simulink model "assignment_2_without_MPPT"  (R2023b)
settings: Solver=VariableStepAuto  StartTime=0.0  StopTime=10  FixedStep=1e-10  MaxStep=1e-4  RelTol=1e-4
values from neighbouring files (symbols this model uses):
  Cdc = 278*10^-3    (= 0.278)    [SOLAR_NEW_MPPT.m]
  fg = 50    [SOLAR_NEW_MPPT.m]
  Ki_cc = Rc/tau_IAC    (= 0.95)    [SOLAR_NEW_MPPT.m]
  Ki_pll = Kp_pll/tau_pll    [SOLAR_NEW_MPPT.m]
  kip = 1/(ki_pq*tau_p)    [SOLAR_NEW_MPPT.m]
  Kiv = w1^2*Cdc    (= 27437.500235)    [SOLAR_NEW_MPPT.m]
  Kp_cc = Lc/tau_IAC    (= 0.03031)    [SOLAR_NEW_MPPT.m]
  Kp_pll = (2*w*e)/Va    [SOLAR_NEW_MPPT.m]
  kpp = tau_IAC/(ki_pq*tau_p)    [SOLAR_NEW_MPPT.m]
  Kpv = 2*e1*w1*Cdc    (= 122.270786078)    [SOLAR_NEW_MPPT.m]
  Lc = 30.31*10^-6    (= 3.031e-05)    [SOLAR_NEW_MPPT.m]
  Rc = 0.95*10^-3    (= 0.00095)    [SOLAR_NEW_MPPT.m]
  Va = sqrt(2)*(Vg/sqrt(3))    [SOLAR_NEW_MPPT.m]
  Vdcn = 1200    [SOLAR_NEW_MPPT.m]
undefined symbols (not defined in the file or in its folder): Io, L, R
libraries: spsControlledVoltageSourceLib x6, slpidlib x6, spsSeriesRLCBranchLib x4, spsControlledCurrentSourceLib x2, spsCurrentMeasurementLib x2, spsGroundLib x1, spsabctodq0Lib x1, spsPower3phInstantaneousLib x1, spsThreePhaseVIMeasurementLib x1, spsVoltageMeasurementLib x1, spspowerguiLib x1
settings Model: Creator=TW  LastModifiedBy=User
settings OptimizationCC: ReuseModelBlockBuffer=off

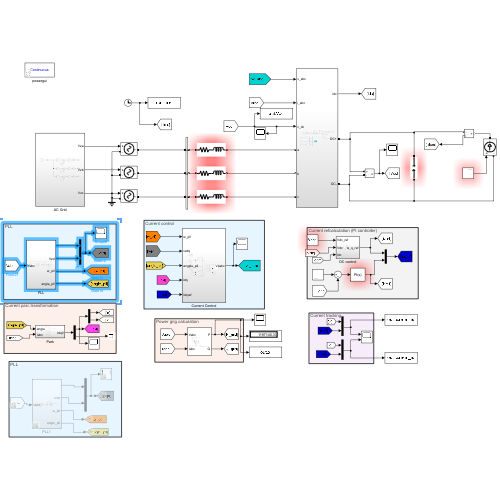
[thumbnail: Simulink's stored preview of the top-level diagram]
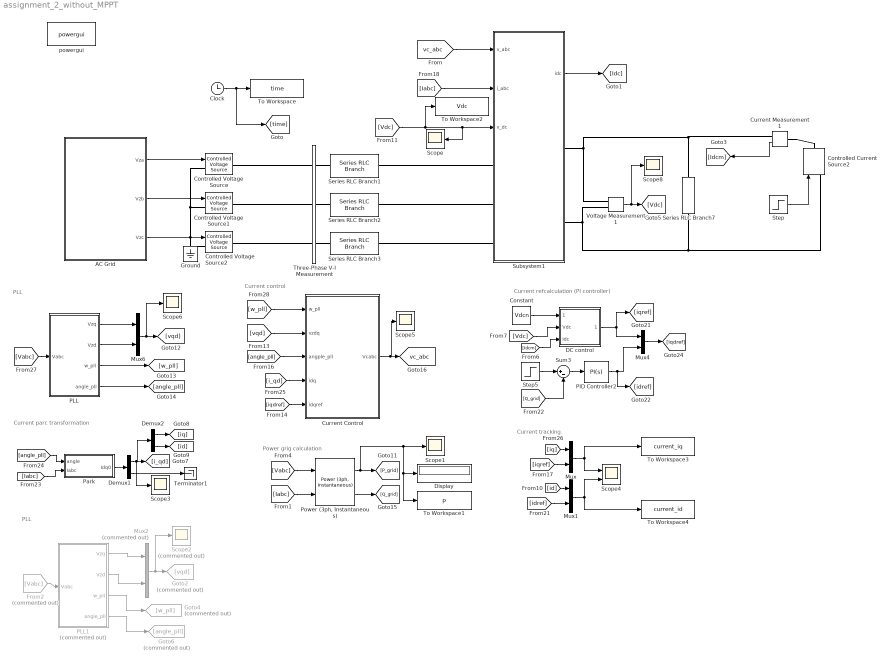
== system assignment_2_without_MPPT ==
  note: Current parc transformation
  note: PLL
  note: Power grig calculation
  note: Current control
  note: Current tracking
  note: Current refcalculation (PI controller)
  note: PLL
  AC Grid : Subsystem
  Clock : Clock
  Constant : Constant  Value=Vdcn
  Controlled Current Source2 : spsControlledCurrentSourceLib/Controlled Current Source  Initialize=on  Source_Type=AC  Amplitude=0  Phase=0  Frequency=0  Measurements=None
  Controlled Voltage Source : spsControlledVoltageSourceLib/Controlled Voltage Source  Initialize=on  Source_Type=AC  Amplitude=0  Phase=0  Frequency=0  Measurements=None
  Controlled Voltage Source1 : spsControlledVoltageSourceLib/Controlled Voltage Source  Initialize=on  Source_Type=AC  Amplitude=0  Phase=0  Frequency=0  Measurements=None
  Controlled Voltage Source2 : spsControlledVoltageSourceLib/Controlled Voltage Source  Initialize=on  Source_Type=AC  Amplitude=0  Phase=0  Frequency=0  Measurements=None
  Current Control : Subsystem
  Current Measurement1 : spsCurrentMeasurementLib/Current Measurement  PhasorSimulation=off  OutputType=Complex  PSBequivalent=0
  DC control : Subsystem
  Demux1 : Demux  Outputs=2
  Demux2 : Demux  Outputs=2
  Display : Display
      settings: Format=bank
  From2 : From  Commented=on  GotoTag=Vabc  TagVisibility=global
  Goto2 : Goto  Commented=on  GotoTag=vqd
  Goto4 : Goto  Commented=on  GotoTag=w_pll
  Goto6 : Goto  Commented=on  GotoTag=angle_pll
  Ground : spsGroundLib/Ground  LConnTagsString=a
  Mux{,1,4,6} (4 alike) : Mux  Inputs=2
  Mux2 : Mux  Commented=on  Inputs=2
  PID Controller2 : slpidlib/PID Controller  Controller=PI  Form=Parallel  TimeDomain=Continuous-time  UseExternalTs=off  SampleTime=-1  IntegratorMethod=Forward Euler  FilterMethod=Forward Euler  ControllerParametersSource=internal  P=kpp  I=kip  UseKiTs=off  D=0  N=100  UseFilter=on  TunerSelectOption=Transfer Function Based (PID Tuner App)  InitialConditionSource=internal  InitialConditionForIntegrator=0  InitialConditionForFilter=0  DifferentiatorICPrevScaledInput=0  ExternalReset=none  TrackingMode=off  Kt=1  LimitOutput=off  SatLimitsSource=internal  UpperSaturationLimit=inf  LowerSaturationLimit=-inf  LinearizeAsGain=on  AntiWindupMode=none  Kb=1  LimitIntegrator=off  UpperIntegratorSaturationLimit=inf  LowerIntegratorSaturationLimit=-inf  POutMin=[]  POutMax=[]  IOutMin=[]  IOutMax=[]  DOutMin=[]  DOutMax=[]  NOutMin=[]  NOutMax=[]  SumOutMin=[]  SumOutMax=[]  SaturationOutMin=[]  SaturationOutMax=[]  PParamMin=[]  PParamMax=[]  IParamMin=[]  IParamMax=[]  DParamMin=[]  DParamMax=[]  NParamMin=[]  NParamMax=[]  KbParamMin=[]  KbParamMax=[]  KtParamMin=[]  KtParamMax=[]  KbOutMin=[]  KbOutMax=[]  KtOutMin=[]  KtOutMax=[]  IntegratorOutMin=[]  IntegratorOutMax=[]  FilterOutMin=[]  FilterOutMax=[]  SumI1OutMin=[]  SumI1OutMax=[]  SumI2OutMin=[]  SumI2OutMax=[]  SumI3OutMin=[]  SumI3OutMax=[]  SumI4OutMin=[]  SumI4OutMax=[]  SumDOutMin=[]  SumDOutMax=[]  DifferentiatorOutMin=[]  DifferentiatorOutMax=[]  FilterDiffOutCoefMin=[]  FilterDiffOutCoefMax=[]  ReciprocalOutMin=[]  ReciprocalOutMax=[]  SumDenOutMin=[]  SumDenOutMax=[]  SumNumOutMin=[]  SumNumOutMax=[]  DivideOutMin=[]  DivideOutMax=[]  UdiffTsProdOutMin=[]  UdiffTsProdOutMax=[]  NTsProdOutMin=[]  NTsProdOutMax=[]  UintegralTsProdOutMin=[]  UintegralTsProdOutMax=[]  UngainTsProdOutMin=[]  UngainTsProdOutMax=[]  ClampingZeroOutDataTypeStr=Inherit: Inherit via back propagation  ClampingZeroOutMin=[]  ClampingZeroOutMax=[]  FilterDenConstantOutDataTypeStr=Inherit: Inherit via back propagation  FilterDenConstantOutMin=[]  FilterDenConstantOutMax=[]  PCopyOutDataTypeStr=Inherit: Inherit via back propagation  PCopyOutMin=[]  PCopyOutMax=[]  NCopyOutDataTypeStr=Inherit: Inherit via back propagation  NCopyOutMin=[]  NCopyOutMax=[]  IntegratorContinuousStateAttributes=''  IntegratorStateMustResolveToSignalObject=off  IntegratorRTWStateStorageClass=Auto  FilterContinuousStateAttributes=''  FilterStateMustResolveToSignalObject=off  FilterRTWStateStorageClass=Auto  ParallelPVariant=InternalParameters  IdealPVariant=Disabled  IVariant=InternalParameters  DVariant=Disabled  IntegratorVariant=Continuous  SatVariant=Disabled  AWVariant=Passthrough  PCopyVariant=Disabled  TRVariant=Disabled  FdbkBlocksVariant=Forward  IdealPFdbkVariant=Disabled  SatFdbkVariant=Disabled  DerivativeFilterVariant=Disabled  NVariant=Disabled  NCopyVariant=Disabled_SignalSpec  FilterICVariant=Disabled  IntegratorICVariant=InternalICs  ExternalResetVariant=Disabled  TRSumVariant=Passthrough  SumFdbkVariant=Disabled  SumVariant=Sum_PI  TsampFilterVariant=InternalTs  TsampNgainVariant=Passthrough  TsampIntegralVariant=Disabled_SignalSpec  ExternalSaturationOutDataTypeStr=Inherit: Same as second input
  PLL : Subsystem
  PLL1 : Subsystem  Commented=on
  Park : Subsystem
  "Power (3ph, Instantaneous)" : spsPower3phInstantaneousLib/Power (3ph, Instantaneous)
  Scope{,1,3,5..6,8} (6 alike) : Scope
  Scope2 : Scope  Commented=on
  Scope4 : Scope  NumInputPorts=2
  Series RLC Branch1 : spsSeriesRLCBranchLib/Series RLC Branch  LConnTagsString=__new0  RConnTagsString=__new0  BranchType=RL  Resistance=Rc  Inductance=Lc  SetiL0=off  InitialCurrent=0  Capacitance=1e-6  Setx0=off  InitialVoltage=0  Measurements=None
  Series RLC Branch2 : spsSeriesRLCBranchLib/Series RLC Branch  LConnTagsString=__new0  RConnTagsString=__new0  BranchType=RL  Resistance=Rc  Inductance=Lc  SetiL0=off  InitialCurrent=0  Capacitance=1e-6  Setx0=off  InitialVoltage=0  Measurements=None
  Series RLC Branch3 : spsSeriesRLCBranchLib/Series RLC Branch  LConnTagsString=__new0  RConnTagsString=__new0  BranchType=RL  Resistance=Rc  Inductance=Lc  SetiL0=off  InitialCurrent=0  Capacitance=1e-6  Setx0=off  InitialVoltage=0  Measurements=None
  Series RLC Branch7 : spsSeriesRLCBranchLib/Series RLC Branch  LConnTagsString=__new0  RConnTagsString=__new0  BranchType=C  Resistance=R  Inductance=L  SetiL0=off  InitialCurrent=0  Capacitance=Cdc  Setx0=on  InitialVoltage=Vdcn  Measurements=None
  Step : Step  After=Io  SampleTime=0
  Step5 : Step  Time=1.5  After=0  SampleTime=0
  Subsystem1 : Subsystem
  Sum3 : Sum  Inputs=|+-
  Terminator1 : Terminator
  Three-Phase V-I Measurement : spsThreePhaseVIMeasurementLib/Three-Phase V-I Measurement  VoltageMeasurement=phase-to-ground  SetLabelV=on  LabelV=Vabc  Vpu=off  VpuLL=off  CurrentMeasurement=yes  SetLabelI=on  LabelI=Iabc  Ipu=off  Pbase=100e6  Vbase=500e3  OutputType=Complex  PhasorSimulation=off  PSBequivalent=0
  To Workspace : ToWorkspace  VariableName=time  SampleTime=-1
  To Workspace1 : ToWorkspace  VariableName=p  SampleTime=-1
  To Workspace2 : ToWorkspace  VariableName=Vdc  SampleTime=-1
  To Workspace3 : ToWorkspace  VariableName=current_iq  SampleTime=-1
  To Workspace4 : ToWorkspace  VariableName=current_id  SampleTime=-1
  Voltage Measurement1 : spsVoltageMeasurementLib/Voltage Measurement  PhasorSimulation=off  OutputType=Complex  PSBequivalent=0
  powergui : spspowerguiLib/powergui  Priority=1  SimulationMode=Continuous  SampleTime=1e-10  frequency=60  Iterations=50  frequencyindice=0  Pbase=100e6  ErrMax=1e-4  UnitsV=kV  UnitsW=MW  buscounter=0  FunctionMessages=off  echomessages=off  EnableUseOfTLC=off  CurrentSourceSwitches=off  DisableSnubberDevices=off  DisableRonSwitches=off  DisableVfSwitches=off  DisplayEquations=off  AutomaticDiscreteSolvers=off  SolverType=Tustin/Backward Euler (TBE)  Interpol=off  ExternalGateDelay=off  methode=off  Ts=100  x0status=blocks  SPID=on  SwTol=0  HookPort=off  NonlinearTolerance=1e-4  nMaxIteration=100  ContinueOnMaxIteration=off  RestoreLinks=warning  ResistiveCurrentMeasurement=off  Frange=[0:2:500]  Ylog=off  Xlog=on  ShowGrid=off  save=off  variable=ZData  structure=0  ZoomFFT=off  StartTime=0.0  cycles=1  DisplayStyle=1  fundamental=60  FreqAxis=off  MaxFrequency=1000  frequencyindicesteady=1  RmsSteady=1  display=off
  tag scope: vc_abc=global
  wires:
  Voltage Measurement1/1 -> Scope8/1, [Vdc]
  Current Measurement1/1 -> [Idcm]
  [Iabc] -> Subsystem1/2(i_abc)
  "Power (3ph, Instantaneous)"/1 -> To Workspace1/1, Display/1, Scope1/1, [P_grid]
  [Vabc] -> "Power (3ph, Instantaneous)"/1
  Demux2/1 -> [iq]
  [angle_pll] -> Current Control/3(angple_pll)
  [i_qd] -> Current Control/4(idq)
  [idref] -> Mux1/2
  [iq] -> Mux/1
  [iqdref] -> Current Control/5(idqref)
  [vqd] -> Current Control/2(vzdq)
  PLL/2(Vzd) -> Mux6/2
  Demux1/1 -> Scope3/1, Demux2/1, [i_qd]
  [iqref] -> Mux/2
  [id] -> Mux1/1
  Demux2/2 -> [id]
  "Power (3ph, Instantaneous)"/2 -> [Q_grid]
  PLL/4(angle_pll) -> [angle_pll]
  [angle_pll] -> Park/1(angle)
  Current Control/1(Vcabc) -> Scope5/1, [vc_abc]
  [w_pll] -> Current Control/1(w_pll)
  Demux1/2 -> Terminator1/1
  [Iabc] -> "Power (3ph, Instantaneous)"/2
  [Iabc] -> Park/2(Iabc)
  Park/1(Idq0) -> Demux1/1
  [Vabc] -> PLL/1(Vabc)
  PLL/1(Vzq) -> Mux6/1
  Mux6/1 -> Scope6/1, [vqd]
  Mux1/1 -> To Workspace4/1, Scope4/2
  PLL/3(w_pll) -> [w_pll]
  Subsystem1/1(idc) -> [Idc]
  [vc_abc] -> Subsystem1/1(v_abc)
  Step/1 -> Controlled Current Source2/1
  [Vdc] -> Subsystem1/3(v_dc), Scope/1, To Workspace2/1
  Clock/1 -> [time], To Workspace/1
  Mux/1 -> To Workspace3/1, Scope4/1
  [Vdc] -> DC control/2(Vdc)
  Sum3/1 -> PID Controller2/1
  Constant/1 -> DC control/1(Vdc_ref)
  [Q_grid] -> Sum3/2
  [Idcm] -> DC control/3(Idc)
  PID Controller2/1 -> [idref], Mux4/2
  Step5/1 -> Sum3/1
  DC control/1(is_q_ref) -> [iqref], Mux4/1
  Mux4/1 -> [iqdref]
  AC Grid/1(Vza) -> Controlled Voltage Source/1
  AC Grid/2(Vzb) -> Controlled Voltage Source1/1
  AC Grid/3(Vzc) -> Controlled Voltage Source2/1
  From2/1 -> PLL1/1(Vabc)
  PLL1/3(w_pll) -> Goto4/1
  PLL1/1(Vzq) -> Mux2/1
  PLL1/2(Vzd) -> Mux2/2
  Mux2/1 -> Scope2/1, Goto2/1
  PLL1/4(angle_pll) -> Goto6/1
  connections:
  Controlled Current Source2/LConn1 -- Subsystem1/RConn2 -- Voltage Measurement1/LConn2 -- Series RLC Branch7/RConn1
  Voltage Measurement1/LConn1 -- Current Measurement1/RConn1 -- Series RLC Branch7/LConn1 -- Subsystem1/RConn1
  Current Measurement1/LConn1 -- Controlled Current Source2/RConn1
  Series RLC Branch1/RConn1 -- Subsystem1/LConn1
  Series RLC Branch3/RConn1 -- Subsystem1/LConn3
  Three-Phase V-I Measurement/LConn3 -- Series RLC Branch3/LConn1
  Series RLC Branch2/RConn1 -- Subsystem1/LConn2
  Three-Phase V-I Measurement/LConn2 -- Series RLC Branch2/LConn1
  Three-Phase V-I Measurement/LConn1 -- Series RLC Branch1/LConn1
  Controlled Voltage Source1/LConn1 -- Controlled Voltage Source/LConn1 -- Controlled Voltage Source2/LConn1 -- Ground/LConn1
  Controlled Voltage Source2/RConn1 -- Three-Phase V-I Measurement/RConn3
  Controlled Voltage Source1/RConn1 -- Three-Phase V-I Measurement/RConn2
  Controlled Voltage Source/RConn1 -- Three-Phase V-I Measurement/RConn1

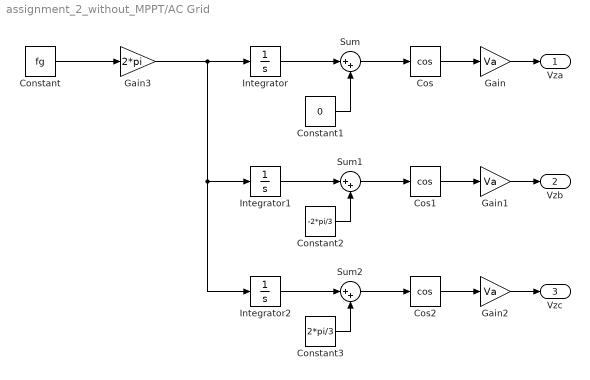
== system assignment_2_without_MPPT/AC Grid ==
  Constant : Constant  Value=fg
  Constant1 : Constant  Value=0
  Constant2 : Constant  Value=-2*pi/3
  Constant3 : Constant  Value=2*pi/3
  Cos : Trigonometry  Operator=cos
  Cos1 : Trigonometry  Operator=cos
  Cos2 : Trigonometry  Operator=cos
  Gain : Gain  Gain=Va
  Gain1 : Gain  Gain=Va
  Gain2 : Gain  Gain=Va
  Gain3 : Gain  Gain=2*pi
  Integrator : Integrator
  Integrator1 : Integrator
  Integrator2 : Integrator
  Sum : Sum  Inputs=|++
  Sum1 : Sum  Inputs=|++
  Sum2 : Sum  Inputs=|++
  Vza : Outport
  Vzb : Outport  Port=2
  Vzc : Outport  Port=3
  wires:
  Integrator2/1 -> Sum2/1
  Cos/1 -> Gain/1
  Gain3/1 -> Integrator1/1, Integrator2/1, Integrator/1
  Integrator1/1 -> Sum1/1
  Cos2/1 -> Gain2/1
  Constant1/1 -> Sum/2
  Gain1/1 -> Vzb/1
  Constant2/1 -> Sum1/2
  Constant3/1 -> Sum2/2
  Gain/1 -> Vza/1
  Sum2/1 -> Cos2/1
  Cos1/1 -> Gain1/1
  Sum/1 -> Cos/1
  Sum1/1 -> Cos1/1
  Gain2/1 -> Vzc/1
  Constant/1 -> Gain3/1
  Integrator/1 -> Sum/1

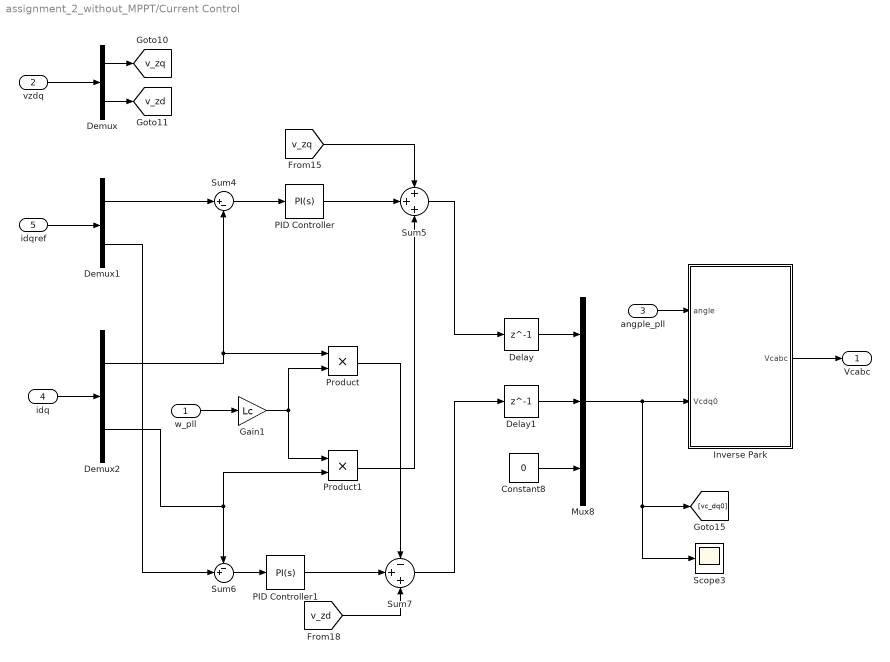
== system assignment_2_without_MPPT/Current Control ==
  w_pll : Inport
  vzdq : Inport  Port=2
  angple_pll : Inport  Port=3
  idq : Inport  Port=4
  idqref : Inport  Port=5
  Constant8 : Constant  Value=0
  Delay : Delay  DelayLength=1
  Delay1 : Delay  DelayLength=1
  Demux : Demux  Outputs=2
  Demux1 : Demux  Outputs=2
  Demux2 : Demux  Outputs=2
  Gain1 : Gain  Gain=Lc
  Inverse Park : Subsystem
  Mux8 : Mux  Inputs=3
  PID Controller : slpidlib/PID Controller  Controller=PI  Form=Parallel  TimeDomain=Continuous-time  UseExternalTs=off  SampleTime=-1  IntegratorMethod=Forward Euler  FilterMethod=Forward Euler  ControllerParametersSource=internal  P=Kp_cc  I=Ki_cc  UseKiTs=off  D=0  N=100  UseFilter=on  TunerSelectOption=Transfer Function Based (PID Tuner App)  InitialConditionSource=internal  InitialConditionForIntegrator=0  InitialConditionForFilter=0  DifferentiatorICPrevScaledInput=0  ExternalReset=none  TrackingMode=off  Kt=1  LimitOutput=off  SatLimitsSource=internal  UpperSaturationLimit=inf  LowerSaturationLimit=-inf  LinearizeAsGain=on  AntiWindupMode=none  Kb=1  LimitIntegrator=off  UpperIntegratorSaturationLimit=inf  LowerIntegratorSaturationLimit=-inf  POutMin=[]  POutMax=[]  IOutMin=[]  IOutMax=[]  DOutMin=[]  DOutMax=[]  NOutMin=[]  NOutMax=[]  SumOutMin=[]  SumOutMax=[]  SaturationOutMin=[]  SaturationOutMax=[]  PParamMin=[]  PParamMax=[]  IParamMin=[]  IParamMax=[]  DParamMin=[]  DParamMax=[]  NParamMin=[]  NParamMax=[]  KbParamMin=[]  KbParamMax=[]  KtParamMin=[]  KtParamMax=[]  KbOutMin=[]  KbOutMax=[]  KtOutMin=[]  KtOutMax=[]  IntegratorOutMin=[]  IntegratorOutMax=[]  FilterOutMin=[]  FilterOutMax=[]  SumI1OutMin=[]  SumI1OutMax=[]  SumI2OutMin=[]  SumI2OutMax=[]  SumI3OutMin=[]  SumI3OutMax=[]  SumI4OutMin=[]  SumI4OutMax=[]  SumDOutMin=[]  SumDOutMax=[]  DifferentiatorOutMin=[]  DifferentiatorOutMax=[]  FilterDiffOutCoefMin=[]  FilterDiffOutCoefMax=[]  ReciprocalOutMin=[]  ReciprocalOutMax=[]  SumDenOutMin=[]  SumDenOutMax=[]  SumNumOutMin=[]  SumNumOutMax=[]  DivideOutMin=[]  DivideOutMax=[]  UdiffTsProdOutMin=[]  UdiffTsProdOutMax=[]  NTsProdOutMin=[]  NTsProdOutMax=[]  UintegralTsProdOutMin=[]  UintegralTsProdOutMax=[]  UngainTsProdOutMin=[]  UngainTsProdOutMax=[]  ClampingZeroOutDataTypeStr=Inherit: Inherit via back propagation  ClampingZeroOutMin=[]  ClampingZeroOutMax=[]  FilterDenConstantOutDataTypeStr=Inherit: Inherit via back propagation  FilterDenConstantOutMin=[]  FilterDenConstantOutMax=[]  PCopyOutDataTypeStr=Inherit: Inherit via back propagation  PCopyOutMin=[]  PCopyOutMax=[]  NCopyOutDataTypeStr=Inherit: Inherit via back propagation  NCopyOutMin=[]  NCopyOutMax=[]  IntegratorContinuousStateAttributes=''  IntegratorStateMustResolveToSignalObject=off  IntegratorRTWStateStorageClass=Auto  FilterContinuousStateAttributes=''  FilterStateMustResolveToSignalObject=off  FilterRTWStateStorageClass=Auto  ParallelPVariant=InternalParameters  IdealPVariant=Disabled  IVariant=InternalParameters  DVariant=Disabled  IntegratorVariant=Continuous  SatVariant=Disabled  AWVariant=Passthrough  PCopyVariant=Disabled  TRVariant=Disabled  FdbkBlocksVariant=Forward  IdealPFdbkVariant=Disabled  SatFdbkVariant=Disabled  DerivativeFilterVariant=Disabled  NVariant=Disabled  NCopyVariant=Disabled_SignalSpec  FilterICVariant=Disabled  IntegratorICVariant=InternalICs  ExternalResetVariant=Disabled  TRSumVariant=Passthrough  SumFdbkVariant=Disabled  SumVariant=Sum_PI  TsampFilterVariant=InternalTs  TsampNgainVariant=Passthrough  TsampIntegralVariant=Disabled_SignalSpec  ExternalSaturationOutDataTypeStr=Inherit: Same as second input
  PID Controller1 : slpidlib/PID Controller  Controller=PI  Form=Parallel  TimeDomain=Continuous-time  UseExternalTs=off  SampleTime=-1  IntegratorMethod=Forward Euler  FilterMethod=Forward Euler  ControllerParametersSource=internal  P=Kp_cc  I=Ki_cc  UseKiTs=off  D=0  N=100  UseFilter=on  TunerSelectOption=Transfer Function Based (PID Tuner App)  InitialConditionSource=internal  InitialConditionForIntegrator=0  InitialConditionForFilter=0  DifferentiatorICPrevScaledInput=0  ExternalReset=none  TrackingMode=off  Kt=1  LimitOutput=off  SatLimitsSource=internal  UpperSaturationLimit=inf  LowerSaturationLimit=-inf  LinearizeAsGain=on  AntiWindupMode=none  Kb=1  LimitIntegrator=off  UpperIntegratorSaturationLimit=inf  LowerIntegratorSaturationLimit=-inf  POutMin=[]  POutMax=[]  IOutMin=[]  IOutMax=[]  DOutMin=[]  DOutMax=[]  NOutMin=[]  NOutMax=[]  SumOutMin=[]  SumOutMax=[]  SaturationOutMin=[]  SaturationOutMax=[]  PParamMin=[]  PParamMax=[]  IParamMin=[]  IParamMax=[]  DParamMin=[]  DParamMax=[]  NParamMin=[]  NParamMax=[]  KbParamMin=[]  KbParamMax=[]  KtParamMin=[]  KtParamMax=[]  KbOutMin=[]  KbOutMax=[]  KtOutMin=[]  KtOutMax=[]  IntegratorOutMin=[]  IntegratorOutMax=[]  FilterOutMin=[]  FilterOutMax=[]  SumI1OutMin=[]  SumI1OutMax=[]  SumI2OutMin=[]  SumI2OutMax=[]  SumI3OutMin=[]  SumI3OutMax=[]  SumI4OutMin=[]  SumI4OutMax=[]  SumDOutMin=[]  SumDOutMax=[]  DifferentiatorOutMin=[]  DifferentiatorOutMax=[]  FilterDiffOutCoefMin=[]  FilterDiffOutCoefMax=[]  ReciprocalOutMin=[]  ReciprocalOutMax=[]  SumDenOutMin=[]  SumDenOutMax=[]  SumNumOutMin=[]  SumNumOutMax=[]  DivideOutMin=[]  DivideOutMax=[]  UdiffTsProdOutMin=[]  UdiffTsProdOutMax=[]  NTsProdOutMin=[]  NTsProdOutMax=[]  UintegralTsProdOutMin=[]  UintegralTsProdOutMax=[]  UngainTsProdOutMin=[]  UngainTsProdOutMax=[]  ClampingZeroOutDataTypeStr=Inherit: Inherit via back propagation  ClampingZeroOutMin=[]  ClampingZeroOutMax=[]  FilterDenConstantOutDataTypeStr=Inherit: Inherit via back propagation  FilterDenConstantOutMin=[]  FilterDenConstantOutMax=[]  PCopyOutDataTypeStr=Inherit: Inherit via back propagation  PCopyOutMin=[]  PCopyOutMax=[]  NCopyOutDataTypeStr=Inherit: Inherit via back propagation  NCopyOutMin=[]  NCopyOutMax=[]  IntegratorContinuousStateAttributes=''  IntegratorStateMustResolveToSignalObject=off  IntegratorRTWStateStorageClass=Auto  FilterContinuousStateAttributes=''  FilterStateMustResolveToSignalObject=off  FilterRTWStateStorageClass=Auto  ParallelPVariant=InternalParameters  IdealPVariant=Disabled  IVariant=InternalParameters  DVariant=Disabled  IntegratorVariant=Continuous  SatVariant=Disabled  AWVariant=Passthrough  PCopyVariant=Disabled  TRVariant=Disabled  FdbkBlocksVariant=Forward  IdealPFdbkVariant=Disabled  SatFdbkVariant=Disabled  DerivativeFilterVariant=Disabled  NVariant=Disabled  NCopyVariant=Disabled_SignalSpec  FilterICVariant=Disabled  IntegratorICVariant=InternalICs  ExternalResetVariant=Disabled  TRSumVariant=Passthrough  SumFdbkVariant=Disabled  SumVariant=Sum_PI  TsampFilterVariant=InternalTs  TsampNgainVariant=Passthrough  TsampIntegralVariant=Disabled_SignalSpec  ExternalSaturationOutDataTypeStr=Inherit: Same as second input
  Product : Product
  Product1 : Product
  Scope3 : Scope
  Sum4 : Sum  Inputs=|+-
  Sum5 : Sum  Inputs=+++
  Sum6 : Sum  Inputs=-+|
  Sum7 : Sum  Inputs=-++
  Vcabc : Outport
  tag scope: v_zd=global, v_zq=global
  wires:
  Demux1/1 -> Sum4/1
  Demux/2 -> [v_zd]
  Sum6/1 -> PID Controller1/1
  PID Controller1/1 -> Sum7/2
  PID Controller/1 -> Sum5/2
  Demux2/1 -> Sum4/2, Product/1
  Mux8/1 -> Scope3/1, [vc_dq0], Inverse Park/2(Vcdq0)
  w_pll/1 -> Gain1/1
  Gain1/1 -> Product1/1, Product/2
  Demux/1 -> [v_zq]
  Demux2/2 -> Sum6/1, Product1/2
  idqref/1 -> Demux1/1
  [v_zd] -> Sum7/3
  Constant8/1 -> Mux8/3
  Demux1/2 -> Sum6/2
  Sum5/1 -> Delay/1
  Delay/1 -> Mux8/1
  [v_zq] -> Sum5/1
  Inverse Park/1(Vcabc) -> Vcabc/1
  Sum4/1 -> PID Controller/1
  Sum7/1 -> Delay1/1
  vzdq/1 -> Demux/1
  Delay1/1 -> Mux8/2
  Product/1 -> Sum7/1
  Product1/1 -> Sum5/3
  angple_pll/1 -> Inverse Park/1(angle)
  idq/1 -> Demux2/1

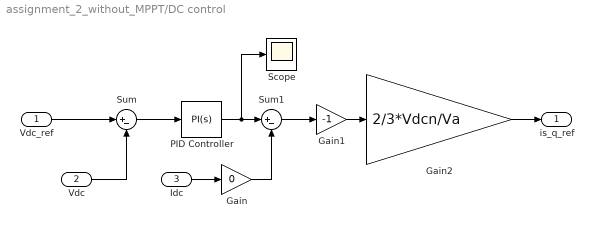
== system assignment_2_without_MPPT/DC control ==
  Vdc_ref : Inport
  Vdc : Inport  Port=2
  Idc : Inport  Port=3
  Gain : Gain  Gain=0
  Gain1 : Gain  Gain=-1
  Gain2 : Gain  Gain=2/3*Vdcn/Va
  PID Controller : slpidlib/PID Controller  Controller=PI  Form=Parallel  TimeDomain=Continuous-time  UseExternalTs=off  SampleTime=-1  IntegratorMethod=Forward Euler  FilterMethod=Forward Euler  ControllerParametersSource=internal  P=Kpv  I=Kiv  UseKiTs=off  D=0  N=100  UseFilter=on  TunerSelectOption=Transfer Function Based (PID Tuner App)  InitialConditionSource=internal  InitialConditionForIntegrator=0  InitialConditionForFilter=0  DifferentiatorICPrevScaledInput=0  ExternalReset=none  TrackingMode=off  Kt=1  LimitOutput=off  SatLimitsSource=internal  UpperSaturationLimit=inf  LowerSaturationLimit=-inf  LinearizeAsGain=on  AntiWindupMode=none  Kb=1  LimitIntegrator=off  UpperIntegratorSaturationLimit=inf  LowerIntegratorSaturationLimit=-inf  POutMin=[]  POutMax=[]  IOutMin=[]  IOutMax=[]  DOutMin=[]  DOutMax=[]  NOutMin=[]  NOutMax=[]  SumOutMin=[]  SumOutMax=[]  SaturationOutMin=[]  SaturationOutMax=[]  PParamMin=[]  PParamMax=[]  IParamMin=[]  IParamMax=[]  DParamMin=[]  DParamMax=[]  NParamMin=[]  NParamMax=[]  KbParamMin=[]  KbParamMax=[]  KtParamMin=[]  KtParamMax=[]  KbOutMin=[]  KbOutMax=[]  KtOutMin=[]  KtOutMax=[]  IntegratorOutMin=[]  IntegratorOutMax=[]  FilterOutMin=[]  FilterOutMax=[]  SumI1OutMin=[]  SumI1OutMax=[]  SumI2OutMin=[]  SumI2OutMax=[]  SumI3OutMin=[]  SumI3OutMax=[]  SumI4OutMin=[]  SumI4OutMax=[]  SumDOutMin=[]  SumDOutMax=[]  DifferentiatorOutMin=[]  DifferentiatorOutMax=[]  FilterDiffOutCoefMin=[]  FilterDiffOutCoefMax=[]  ReciprocalOutMin=[]  ReciprocalOutMax=[]  SumDenOutMin=[]  SumDenOutMax=[]  SumNumOutMin=[]  SumNumOutMax=[]  DivideOutMin=[]  DivideOutMax=[]  UdiffTsProdOutMin=[]  UdiffTsProdOutMax=[]  NTsProdOutMin=[]  NTsProdOutMax=[]  UintegralTsProdOutMin=[]  UintegralTsProdOutMax=[]  UngainTsProdOutMin=[]  UngainTsProdOutMax=[]  ClampingZeroOutDataTypeStr=Inherit: Inherit via back propagation  ClampingZeroOutMin=[]  ClampingZeroOutMax=[]  FilterDenConstantOutDataTypeStr=Inherit: Inherit via back propagation  FilterDenConstantOutMin=[]  FilterDenConstantOutMax=[]  PCopyOutDataTypeStr=Inherit: Inherit via back propagation  PCopyOutMin=[]  PCopyOutMax=[]  NCopyOutDataTypeStr=Inherit: Inherit via back propagation  NCopyOutMin=[]  NCopyOutMax=[]  IntegratorContinuousStateAttributes=''  IntegratorStateMustResolveToSignalObject=off  IntegratorRTWStateStorageClass=Auto  FilterContinuousStateAttributes=''  FilterStateMustResolveToSignalObject=off  FilterRTWStateStorageClass=Auto  ParallelPVariant=InternalParameters  IdealPVariant=Disabled  IVariant=InternalParameters  DVariant=Disabled  IntegratorVariant=Continuous  SatVariant=Disabled  AWVariant=Passthrough  PCopyVariant=Disabled  TRVariant=Disabled  FdbkBlocksVariant=Forward  IdealPFdbkVariant=Disabled  SatFdbkVariant=Disabled  DerivativeFilterVariant=Disabled  NVariant=Disabled  NCopyVariant=Disabled_SignalSpec  FilterICVariant=Disabled  IntegratorICVariant=InternalICs  ExternalResetVariant=Disabled  TRSumVariant=Passthrough  SumFdbkVariant=Disabled  SumVariant=Sum_PI  TsampFilterVariant=InternalTs  TsampNgainVariant=Passthrough  TsampIntegralVariant=Disabled_SignalSpec  ExternalSaturationOutDataTypeStr=Inherit: Same as second input
  Scope : Scope
  Sum : Sum  Inputs=|+-
  Sum1 : Sum  Inputs=|+-
  is_q_ref : Outport
  wires:
  Gain2/1 -> is_q_ref/1
  Sum1/1 -> Gain1/1
  Sum/1 -> PID Controller/1
  Gain1/1 -> Gain2/1
  Gain/1 -> Sum1/2
  Vdc_ref/1 -> Sum/1
  PID Controller/1 -> Sum1/1, Scope/1
  Vdc/1 -> Sum/2
  Idc/1 -> Gain/1

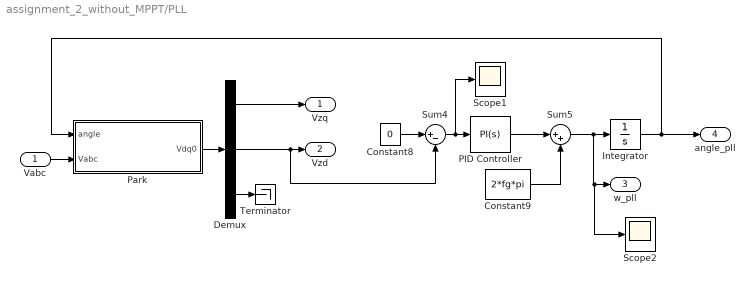
== system assignment_2_without_MPPT/PLL ==
  Vabc : Inport
  Constant8 : Constant  Value=0
  Constant9 : Constant  Value=2*fg*pi
  Demux : Demux  Outputs=3
  Integrator : Integrator
  PID Controller : slpidlib/PID Controller  Controller=PI  Form=Parallel  TimeDomain=Continuous-time  UseExternalTs=off  SampleTime=-1  IntegratorMethod=Forward Euler  FilterMethod=Forward Euler  ControllerParametersSource=internal  P=Kp_pll  I=Ki_pll  UseKiTs=off  D=0  N=100  UseFilter=on  TunerSelectOption=Transfer Function Based (PID Tuner App)  InitialConditionSource=internal  InitialConditionForIntegrator=0  InitialConditionForFilter=0  DifferentiatorICPrevScaledInput=0  ExternalReset=none  TrackingMode=off  Kt=1  LimitOutput=off  SatLimitsSource=internal  UpperSaturationLimit=inf  LowerSaturationLimit=-inf  LinearizeAsGain=on  AntiWindupMode=none  Kb=1  LimitIntegrator=off  UpperIntegratorSaturationLimit=inf  LowerIntegratorSaturationLimit=-inf  POutMin=[]  POutMax=[]  IOutMin=[]  IOutMax=[]  DOutMin=[]  DOutMax=[]  NOutMin=[]  NOutMax=[]  SumOutMin=[]  SumOutMax=[]  SaturationOutMin=[]  SaturationOutMax=[]  PParamMin=[]  PParamMax=[]  IParamMin=[]  IParamMax=[]  DParamMin=[]  DParamMax=[]  NParamMin=[]  NParamMax=[]  KbParamMin=[]  KbParamMax=[]  KtParamMin=[]  KtParamMax=[]  KbOutMin=[]  KbOutMax=[]  KtOutMin=[]  KtOutMax=[]  IntegratorOutMin=[]  IntegratorOutMax=[]  FilterOutMin=[]  FilterOutMax=[]  SumI1OutMin=[]  SumI1OutMax=[]  SumI2OutMin=[]  SumI2OutMax=[]  SumI3OutMin=[]  SumI3OutMax=[]  SumI4OutMin=[]  SumI4OutMax=[]  SumDOutMin=[]  SumDOutMax=[]  DifferentiatorOutMin=[]  DifferentiatorOutMax=[]  FilterDiffOutCoefMin=[]  FilterDiffOutCoefMax=[]  ReciprocalOutMin=[]  ReciprocalOutMax=[]  SumDenOutMin=[]  SumDenOutMax=[]  SumNumOutMin=[]  SumNumOutMax=[]  DivideOutMin=[]  DivideOutMax=[]  UdiffTsProdOutMin=[]  UdiffTsProdOutMax=[]  NTsProdOutMin=[]  NTsProdOutMax=[]  UintegralTsProdOutMin=[]  UintegralTsProdOutMax=[]  UngainTsProdOutMin=[]  UngainTsProdOutMax=[]  ClampingZeroOutDataTypeStr=Inherit: Inherit via back propagation  ClampingZeroOutMin=[]  ClampingZeroOutMax=[]  FilterDenConstantOutDataTypeStr=Inherit: Inherit via back propagation  FilterDenConstantOutMin=[]  FilterDenConstantOutMax=[]  PCopyOutDataTypeStr=Inherit: Inherit via back propagation  PCopyOutMin=[]  PCopyOutMax=[]  NCopyOutDataTypeStr=Inherit: Inherit via back propagation  NCopyOutMin=[]  NCopyOutMax=[]  IntegratorContinuousStateAttributes=''  IntegratorStateMustResolveToSignalObject=off  IntegratorRTWStateStorageClass=Auto  FilterContinuousStateAttributes=''  FilterStateMustResolveToSignalObject=off  FilterRTWStateStorageClass=Auto  ParallelPVariant=InternalParameters  IdealPVariant=Disabled  IVariant=InternalParameters  DVariant=Disabled  IntegratorVariant=Continuous  SatVariant=Disabled  AWVariant=Passthrough  PCopyVariant=Disabled  TRVariant=Disabled  FdbkBlocksVariant=Forward  IdealPFdbkVariant=Disabled  SatFdbkVariant=Disabled  DerivativeFilterVariant=Disabled  NVariant=Disabled  NCopyVariant=Disabled_SignalSpec  FilterICVariant=Disabled  IntegratorICVariant=InternalICs  ExternalResetVariant=Disabled  TRSumVariant=Passthrough  SumFdbkVariant=Disabled  SumVariant=Sum_PI  TsampFilterVariant=InternalTs  TsampNgainVariant=Passthrough  TsampIntegralVariant=Disabled_SignalSpec  ExternalSaturationOutDataTypeStr=Inherit: Same as second input
  Park : Subsystem
  Scope1 : Scope
  Scope2 : Scope
  Sum4 : Sum  Inputs=|+-
  Sum5 : Sum  Inputs=|++
  Terminator : Terminator
  Vzq : Outport
  Vzd : Outport  Port=2
  w_pll : Outport  Port=3
  angle_pll : Outport  Port=4
  wires:
  Vabc/1 -> Park/2(Vabc)
  Constant8/1 -> Sum4/1
  Demux/2 -> Sum4/2, Vzd/1
  PID Controller/1 -> Sum5/1
  Demux/1 -> Vzq/1
  Park/1(Vdq0) -> Demux/1
  Constant9/1 -> Sum5/2
  Integrator/1 -> angle_pll/1, Park/1(angle)
  Demux/3 -> Terminator/1
  Sum5/1 -> Scope2/1, w_pll/1, Integrator/1
  Sum4/1 -> Scope1/1, PID Controller/1

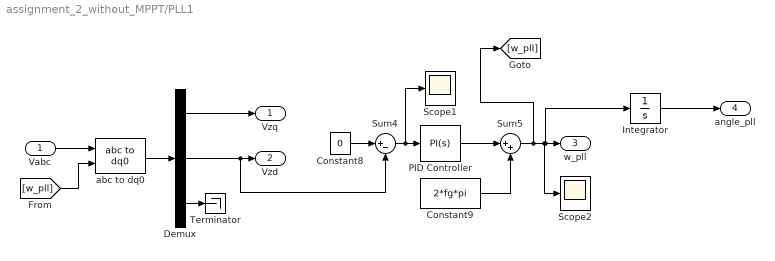
== system assignment_2_without_MPPT/PLL1 ==
  Vabc : Inport
  Constant8 : Constant  Value=0
  Constant9 : Constant  Value=2*fg*pi
  Demux : Demux  Outputs=3
  Integrator : Integrator
  PID Controller : slpidlib/PID Controller  Controller=PI  Form=Parallel  TimeDomain=Continuous-time  UseExternalTs=off  SampleTime=-1  IntegratorMethod=Forward Euler  FilterMethod=Forward Euler  ControllerParametersSource=internal  P=Kp_pll  I=Ki_pll  UseKiTs=off  D=0  N=100  UseFilter=on  TunerSelectOption=Transfer Function Based (PID Tuner App)  InitialConditionSource=internal  InitialConditionForIntegrator=0  InitialConditionForFilter=0  DifferentiatorICPrevScaledInput=0  ExternalReset=none  TrackingMode=off  Kt=1  LimitOutput=off  SatLimitsSource=internal  UpperSaturationLimit=inf  LowerSaturationLimit=-inf  LinearizeAsGain=on  AntiWindupMode=none  Kb=1  LimitIntegrator=off  UpperIntegratorSaturationLimit=inf  LowerIntegratorSaturationLimit=-inf  POutMin=[]  POutMax=[]  IOutMin=[]  IOutMax=[]  DOutMin=[]  DOutMax=[]  NOutMin=[]  NOutMax=[]  SumOutMin=[]  SumOutMax=[]  SaturationOutMin=[]  SaturationOutMax=[]  PParamMin=[]  PParamMax=[]  IParamMin=[]  IParamMax=[]  DParamMin=[]  DParamMax=[]  NParamMin=[]  NParamMax=[]  KbParamMin=[]  KbParamMax=[]  KtParamMin=[]  KtParamMax=[]  KbOutMin=[]  KbOutMax=[]  KtOutMin=[]  KtOutMax=[]  IntegratorOutMin=[]  IntegratorOutMax=[]  FilterOutMin=[]  FilterOutMax=[]  SumI1OutMin=[]  SumI1OutMax=[]  SumI2OutMin=[]  SumI2OutMax=[]  SumI3OutMin=[]  SumI3OutMax=[]  SumI4OutMin=[]  SumI4OutMax=[]  SumDOutMin=[]  SumDOutMax=[]  DifferentiatorOutMin=[]  DifferentiatorOutMax=[]  FilterDiffOutCoefMin=[]  FilterDiffOutCoefMax=[]  ReciprocalOutMin=[]  ReciprocalOutMax=[]  SumDenOutMin=[]  SumDenOutMax=[]  SumNumOutMin=[]  SumNumOutMax=[]  DivideOutMin=[]  DivideOutMax=[]  UdiffTsProdOutMin=[]  UdiffTsProdOutMax=[]  NTsProdOutMin=[]  NTsProdOutMax=[]  UintegralTsProdOutMin=[]  UintegralTsProdOutMax=[]  UngainTsProdOutMin=[]  UngainTsProdOutMax=[]  ClampingZeroOutDataTypeStr=Inherit: Inherit via back propagation  ClampingZeroOutMin=[]  ClampingZeroOutMax=[]  FilterDenConstantOutDataTypeStr=Inherit: Inherit via back propagation  FilterDenConstantOutMin=[]  FilterDenConstantOutMax=[]  PCopyOutDataTypeStr=Inherit: Inherit via back propagation  PCopyOutMin=[]  PCopyOutMax=[]  NCopyOutDataTypeStr=Inherit: Inherit via back propagation  NCopyOutMin=[]  NCopyOutMax=[]  IntegratorContinuousStateAttributes=''  IntegratorStateMustResolveToSignalObject=off  IntegratorRTWStateStorageClass=Auto  FilterContinuousStateAttributes=''  FilterStateMustResolveToSignalObject=off  FilterRTWStateStorageClass=Auto  ParallelPVariant=InternalParameters  IdealPVariant=Disabled  IVariant=InternalParameters  DVariant=Disabled  IntegratorVariant=Continuous  SatVariant=Disabled  AWVariant=Passthrough  PCopyVariant=Disabled  TRVariant=Disabled  FdbkBlocksVariant=Forward  IdealPFdbkVariant=Disabled  SatFdbkVariant=Disabled  DerivativeFilterVariant=Disabled  NVariant=Disabled  NCopyVariant=Disabled_SignalSpec  FilterICVariant=Disabled  IntegratorICVariant=InternalICs  ExternalResetVariant=Disabled  TRSumVariant=Passthrough  SumFdbkVariant=Disabled  SumVariant=Sum_PI  TsampFilterVariant=InternalTs  TsampNgainVariant=Passthrough  TsampIntegralVariant=Disabled_SignalSpec  ExternalSaturationOutDataTypeStr=Inherit: Same as second input
  Scope1 : Scope
  Scope2 : Scope
  Sum4 : Sum  Inputs=|+-
  Sum5 : Sum  Inputs=|++
  Terminator : Terminator
  abc to dq0 : spsabctodq0Lib/abc to dq0  Alignment=90 degrees behind phase A axis
  Vzq : Outport
  Vzd : Outport  Port=2
  w_pll : Outport  Port=3
  angle_pll : Outport  Port=4
  wires:
  Vabc/1 -> abc to dq0/1
  Constant8/1 -> Sum4/1
  Demux/2 -> Sum4/2, Vzd/1
  PID Controller/1 -> Sum5/1
  Demux/1 -> Vzq/1
  abc to dq0/1 -> Demux/1
  Constant9/1 -> Sum5/2
  Demux/3 -> Terminator/1
  Sum5/1 -> [w_pll], Scope2/1, Integrator/1, w_pll/1
  Sum4/1 -> Scope1/1, PID Controller/1
  [w_pll] -> abc to dq0/2
  Integrator/1 -> angle_pll/1

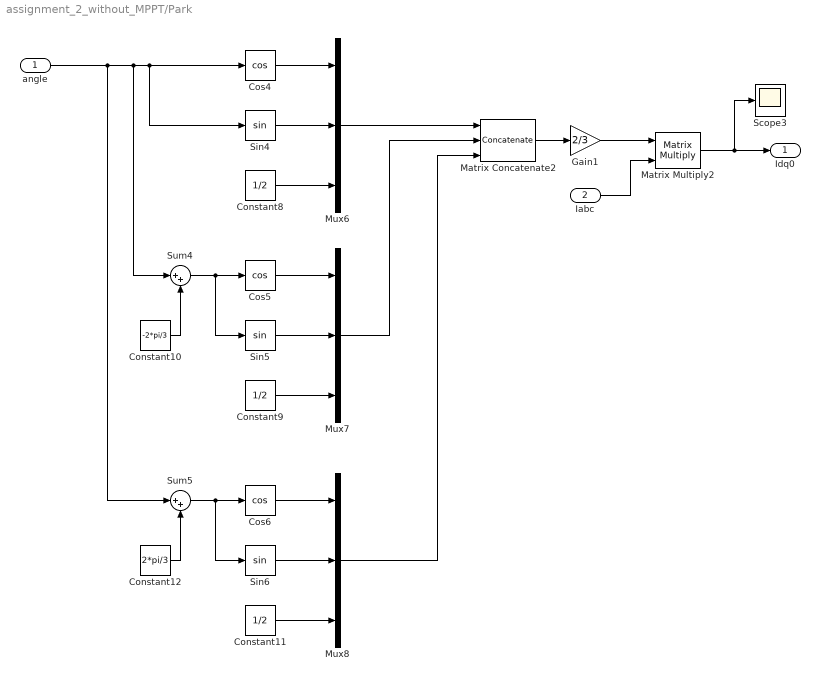
== system assignment_2_without_MPPT/Park ==
  angle : Inport
  Iabc : Inport  Port=2
  Constant10 : Constant  Value=-2*pi/3
  Constant11 : Constant  Value=1/2
  Constant12 : Constant  Value=2*pi/3
  Constant8 : Constant  Value=1/2
  Constant9 : Constant  Value=1/2
  Cos4 : Trigonometry  Operator=cos
  Cos5 : Trigonometry  Operator=cos
  Cos6 : Trigonometry  Operator=cos
  Gain1 : Gain  Gain=2/3
  Matrix Concatenate2 : Concatenate  NumInputs=3  Mode=Multidimensional array  ConcatenateDimension=2
  Matrix Multiply2 : Product  Multiplication=Matrix(*)
  Mux6 : Mux  Inputs=3
  Mux7 : Mux  Inputs=3
  Mux8 : Mux  Inputs=3
  Scope3 : Scope
  Sin4 : Trigonometry
  Sin5 : Trigonometry
  Sin6 : Trigonometry
  Sum4 : Sum  Inputs=|++
  Sum5 : Sum  Inputs=|++
  Idq0 : Outport
  wires:
  angle/1 -> Sum5/1, Sum4/1, Sin4/1, Cos4/1
  Cos5/1 -> Mux7/1
  Mux8/1 -> Matrix Concatenate2/3
  Mux7/1 -> Matrix Concatenate2/2
  Sin6/1 -> Mux8/2
  Sum4/1 -> Sin5/1, Cos5/1
  Iabc/1 -> Matrix Multiply2/2
  Mux6/1 -> Matrix Concatenate2/1
  Constant8/1 -> Mux6/3
  Sum5/1 -> Sin6/1, Cos6/1
  Matrix Multiply2/1 -> Idq0/1, Scope3/1
  Gain1/1 -> Matrix Multiply2/1
  Constant10/1 -> Sum4/2
  Cos4/1 -> Mux6/1
  Sin4/1 -> Mux6/2
  Constant12/1 -> Sum5/2
  Matrix Concatenate2/1 -> Gain1/1
  Constant9/1 -> Mux7/3
  Cos6/1 -> Mux8/1
  Constant11/1 -> Mux8/3
  Sin5/1 -> Mux7/2

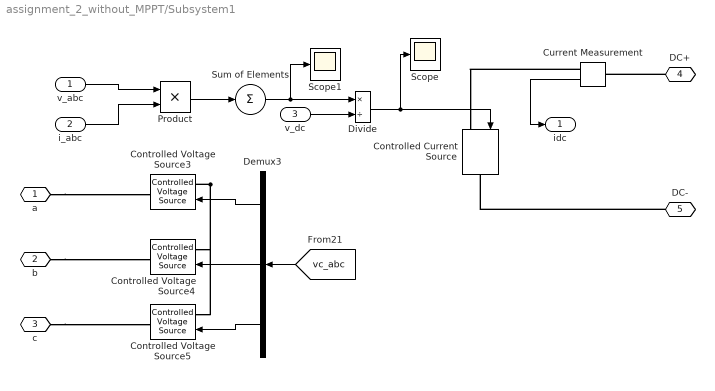
== system assignment_2_without_MPPT/Subsystem1 ==
  v_abc : Inport
  i_abc : Inport  Port=2
  v_dc : Inport  Port=3
  Controlled Current Source : spsControlledCurrentSourceLib/Controlled Current Source  Initialize=on  Source_Type=AC  Amplitude=0  Phase=0  Frequency=0  Measurements=None
  Controlled Voltage Source3 : spsControlledVoltageSourceLib/Controlled Voltage Source  Initialize=on  Source_Type=AC  Amplitude=0  Phase=0  Frequency=0  Measurements=None
  Controlled Voltage Source4 : spsControlledVoltageSourceLib/Controlled Voltage Source  Initialize=on  Source_Type=AC  Amplitude=0  Phase=0  Frequency=0  Measurements=None
  Controlled Voltage Source5 : spsControlledVoltageSourceLib/Controlled Voltage Source  Initialize=on  Source_Type=AC  Amplitude=0  Phase=0  Frequency=0  Measurements=None
  Current Measurement : spsCurrentMeasurementLib/Current Measurement  PhasorSimulation=off  OutputType=Complex  PSBequivalent=0
  Demux3 : Demux  Outputs=3
  Divide : Product  Inputs=*/
  Product : Product
  Scope : Scope
  Scope1 : Scope
  Sum of Elements : Sum  Inputs=+
  a : PMIOPort  Side=Left
  b : PMIOPort  Port=2  Side=Left
  c : PMIOPort  Port=3  Side=Left
  DC+ : PMIOPort  Port=4  Side=Right
  DC- : PMIOPort  Port=5  Side=Right
  idc : Outport
  wires:
  [vc_abc] -> Demux3/1
  Demux3/3 -> Controlled Voltage Source5/1
  Demux3/1 -> Controlled Voltage Source3/1
  Demux3/2 -> Controlled Voltage Source4/1
  v_abc/1 -> Product/1
  i_abc/1 -> Product/2
  Product/1 -> Sum of Elements/1
  Sum of Elements/1 -> Scope1/1, Divide/1
  v_dc/1 -> Divide/2
  Divide/1 -> Scope/1, Controlled Current Source/1
  Current Measurement/1 -> idc/1
  connections:
  Controlled Voltage Source3/LConn1 -- Controlled Voltage Source4/LConn1 -- Controlled Voltage Source5/LConn1
  c/RConn1 -- Controlled Voltage Source5/RConn1
  b/RConn1 -- Controlled Voltage Source4/RConn1
  a/RConn1 -- Controlled Voltage Source3/RConn1
  Current Measurement/RConn1 -- Controlled Current Source/LConn1
  DC+/RConn1 -- Current Measurement/LConn1
  DC-/RConn1 -- Controlled Current Source/RConn1

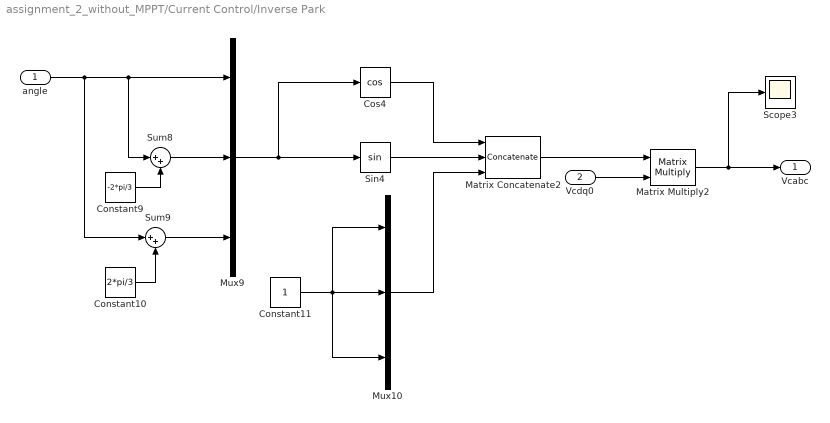
== system assignment_2_without_MPPT/Current Control/Inverse Park ==
  angle : Inport
  Vcdq0 : Inport  Port=2
  Constant10 : Constant  Value=2*pi/3
  Constant11 : Constant
  Constant9 : Constant  Value=-2*pi/3
  Cos4 : Trigonometry  Operator=cos
  Matrix Concatenate2 : Concatenate  NumInputs=3  Mode=Multidimensional array  ConcatenateDimension=2
  Matrix Multiply2 : Product  Multiplication=Matrix(*)
  Mux10 : Mux  Inputs=3
  Mux9 : Mux  Inputs=3
  Scope3 : Scope
  Sin4 : Trigonometry
  Sum8 : Sum  Inputs=|++
  Sum9 : Sum  Inputs=|++
  Vcabc : Outport
  wires:
  Constant11/1 -> Mux10/3, Mux10/1, Mux10/2
  Matrix Multiply2/1 -> Vcabc/1, Scope3/1
  Vcdq0/1 -> Matrix Multiply2/2
  Mux9/1 -> Sin4/1, Cos4/1
  angle/1 -> Sum9/1, Sum8/1, Mux9/1
  Sum9/1 -> Mux9/3
  Matrix Concatenate2/1 -> Matrix Multiply2/1
  Constant10/1 -> Sum9/2
  Cos4/1 -> Matrix Concatenate2/1
  Constant9/1 -> Sum8/2
  Mux10/1 -> Matrix Concatenate2/3
  Sin4/1 -> Matrix Concatenate2/2
  Sum8/1 -> Mux9/2

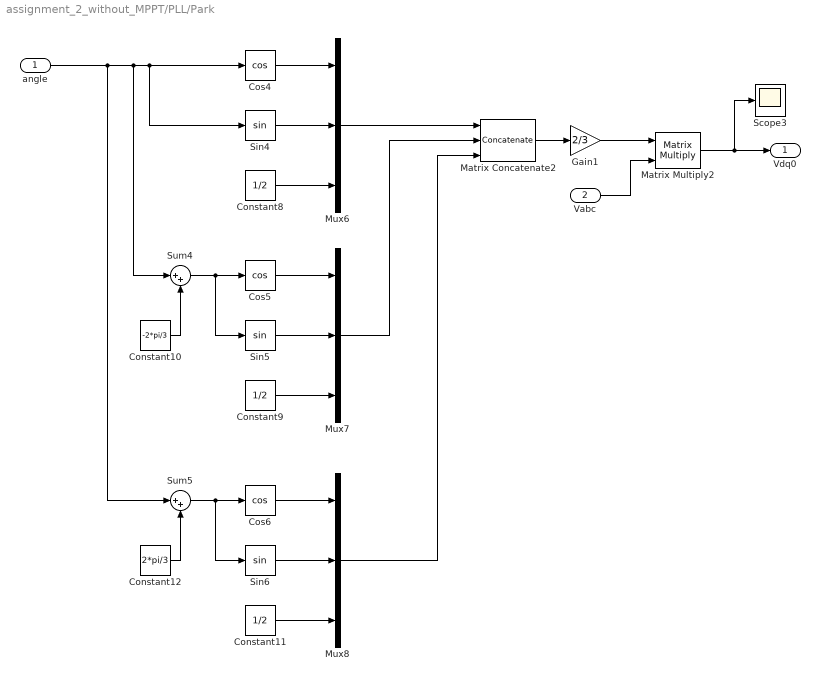
== system assignment_2_without_MPPT/PLL/Park ==
  angle : Inport
  Vabc : Inport  Port=2
  Constant10 : Constant  Value=-2*pi/3
  Constant11 : Constant  Value=1/2
  Constant12 : Constant  Value=2*pi/3
  Constant8 : Constant  Value=1/2
  Constant9 : Constant  Value=1/2
  Cos4 : Trigonometry  Operator=cos
  Cos5 : Trigonometry  Operator=cos
  Cos6 : Trigonometry  Operator=cos
  Gain1 : Gain  Gain=2/3
  Matrix Concatenate2 : Concatenate  NumInputs=3  Mode=Multidimensional array  ConcatenateDimension=2
  Matrix Multiply2 : Product  Multiplication=Matrix(*)
  Mux6 : Mux  Inputs=3
  Mux7 : Mux  Inputs=3
  Mux8 : Mux  Inputs=3
  Scope3 : Scope
  Sin4 : Trigonometry
  Sin5 : Trigonometry
  Sin6 : Trigonometry
  Sum4 : Sum  Inputs=|++
  Sum5 : Sum  Inputs=|++
  Vdq0 : Outport
  wires:
  angle/1 -> Sum5/1, Sum4/1, Sin4/1, Cos4/1
  Cos5/1 -> Mux7/1
  Mux8/1 -> Matrix Concatenate2/3
  Mux7/1 -> Matrix Concatenate2/2
  Sin6/1 -> Mux8/2
  Sum4/1 -> Sin5/1, Cos5/1
  Vabc/1 -> Matrix Multiply2/2
  Mux6/1 -> Matrix Concatenate2/1
  Constant8/1 -> Mux6/3
  Sum5/1 -> Sin6/1, Cos6/1
  Matrix Multiply2/1 -> Vdq0/1, Scope3/1
  Gain1/1 -> Matrix Multiply2/1
  Constant10/1 -> Sum4/2
  Cos4/1 -> Mux6/1
  Sin4/1 -> Mux6/2
  Constant12/1 -> Sum5/2
  Matrix Concatenate2/1 -> Gain1/1
  Constant9/1 -> Mux7/3
  Cos6/1 -> Mux8/1
  Constant11/1 -> Mux8/3
  Sin5/1 -> Mux7/2
